simulink model "calcAttchPtStates_th"  (R2018b)
settings: Solver=VariableStepAuto  StartTime=0.0  StopTime=0  RelTol=1e-3
undefined symbols (not defined in the file): angVel_test, euler_test, pos_test, vel_test
libraries: calcAttchPtStates_ul x1
settings Model: Creator=asiddiq2  LastModifiedBy=asiddiq2

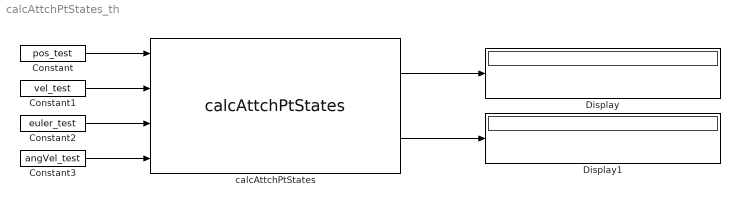
== system calcAttchPtStates_th ==
  Constant : Constant  Value=pos_test
  Constant1 : Constant  Value=vel_test
  Constant2 : Constant  Value=euler_test
  Constant3 : Constant  Value=angVel_test
  Display : Display
  Display1 : Display
  calcAttchPtStates : calcAttchPtStates_ul/calcAttchPtStates  cls_obj=some_class
  wires:
  Constant/1 -> calcAttchPtStates/1
  Constant1/1 -> calcAttchPtStates/2
  Constant2/1 -> calcAttchPtStates/3
  Constant3/1 -> calcAttchPtStates/4
  calcAttchPtStates/1 -> Display/1
  calcAttchPtStates/2 -> Display1/1
